simulink model "sampleModel276"  (R2021b)
settings: Solver=VariableStepAuto  StartTime=0.0  StopTime=10.0  RelTol=1e-3
undefined symbols (not defined in the file or in its folder): magnitude
libraries: simulink x8
settings Model: Creator=user  LastModifiedBy=user

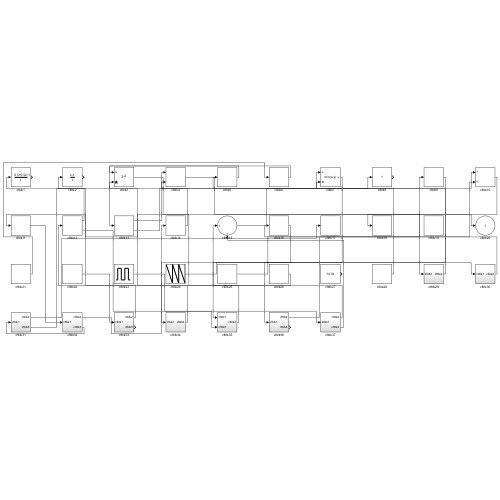
[thumbnail: Simulink's stored preview of the top-level diagram]
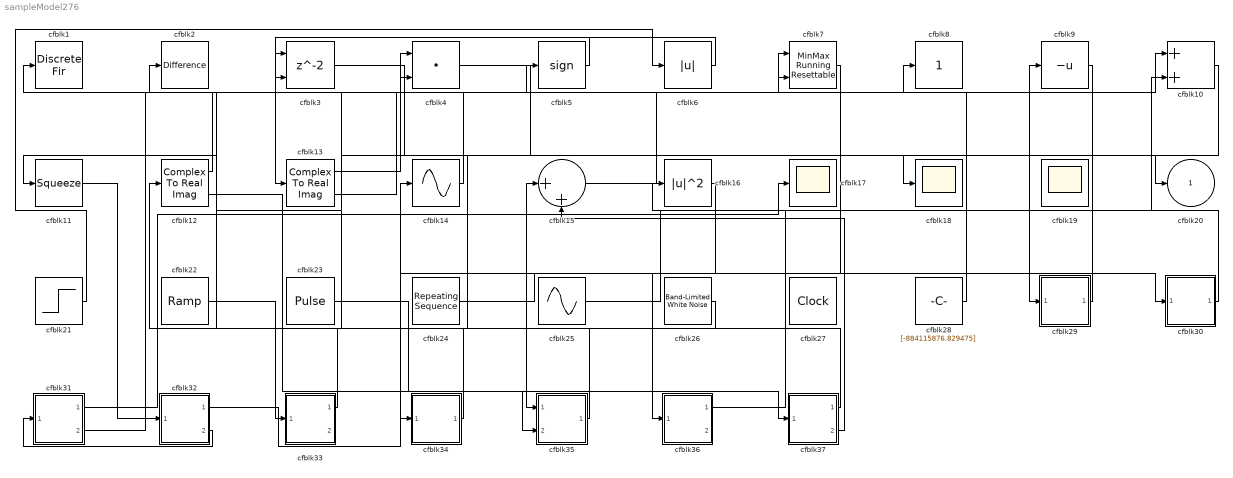
== system sampleModel276 ==
  cfblk1 : DiscreteFir  SampleTime=1
  cfblk10 : Sum
  cfblk11 : Squeeze
  cfblk12 : ComplexToRealImag
  cfblk13 : ComplexToRealImag
  cfblk14 : Sin  TimeSource=Use external signal  SampleTime=0
  cfblk15 : Sum  Inputs=|++
  cfblk16 : Math  Operator=magnitude^2  SaturateOnIntegerOverflow=on
  cfblk17 : Scope
  cfblk18 : Scope
  cfblk19 : Scope
      settings: Floating=on
  cfblk2 : simulink/Discrete/Difference  ICPrevInput=0.0  OutMin=[]  OutMax=[]  OutDataTypeStr=Inherit: Inherit via back propagation  OutDataType=fixdt(1, 16)  OutScaling=2^-10  DoSatur=off
  cfblk21 : Step  Time=[42.000000]  Before=[818983502.483932]  After=[406808043.448474]  SampleTime=0
  cfblk22 : simulink/Sources/Ramp  slope=[-5921.326981]  start=[18.629746]  InitialOutput=[471851.470931]
  cfblk23 : DiscretePulseGenerator  PulseType=Time based  Amplitude=[324430703.930867]  Period=[32077429.850267]  PulseWidth=5  PhaseDelay=[1.000000]
  cfblk24 : simulink/Sources/Repeating Sequence  rep_seq_t=[0 2]  rep_seq_y=[318550818.027670, -776199199.339389]
  cfblk25 : Sin  Amplitude=[-915052577.829016]  Bias=[110707701.179518]  SampleTime=0
  cfblk26 : simulink/Sources/Band-Limited White Noise  Cov=[1529198104.316618]  Ts=0.1  seed=[8998579726.000000]
  cfblk27 : DigitalClock
  cfblk28 : Constant  Value=[-884115876.829475]  SampleTime=1
  cfblk29 : Subsystem
  cfblk3 : Delay  ShowEnablePort=on  SampleTime=1
      settings: InputPortMap=u0,e6
  cfblk30 : Subsystem
  cfblk31 : Subsystem
  cfblk32 : Subsystem
  cfblk33 : Subsystem
  cfblk34 : Subsystem
  cfblk35 : Subsystem
  cfblk36 : Subsystem
  cfblk37 : Subsystem
  cfblk4 : DotProduct  InputSameDT=on  OutDataTypeStr=Inherit: Inherit via internal rule
  cfblk5 : Signum
  cfblk6 : Abs
  cfblk7 : simulink/Math Operations/MinMax Running Resettable  Function=min  vinit=0.0
  cfblk8 : simulink/Math Operations/Slider Gain  gain=1  low=0  high=2
  cfblk9 : UnaryMinus
  cfblk20 : Outport
  wires:
  cfblk4/1 -> cfblk20/1
  cfblk15/1 -> cfblk7/1
  cfblk25/1 -> cfblk9/1
  cfblk5/1 -> cfblk13/1
  cfblk33/1(cfblk2) -> cfblk12/1
  cfblk29/1(cfblk2) -> cfblk7/2
  cfblk32/1(cfblk2) -> cfblk14/1
  cfblk23/1 -> cfblk37/1(cfblk1)
  cfblk26/1 -> cfblk11/1
  cfblk11/1 -> cfblk32/1(cfblk1)
  cfblk12/1 -> cfblk1/1
  cfblk22/1 -> cfblk33/1(cfblk1)
  cfblk32/2(cfblk3) -> cfblk31/1(cfblk1)
  cfblk3/1 -> cfblk29/1(cfblk1)
  cfblk13/1 -> cfblk4/1
  cfblk13/2 -> cfblk10/1
  cfblk37/1(cfblk2) -> cfblk15/1
  cfblk24/1 -> cfblk30/1(cfblk1)
  cfblk21/1 -> cfblk6/1
  cfblk34/1(cfblk2) -> cfblk2/1
  cfblk31/1(cfblk2) -> cfblk17/1
  cfblk16/1 -> cfblk34/1(cfblk1)
  cfblk28/1 -> cfblk5/1
  cfblk14/1 -> cfblk4/2
  cfblk31/2(cfblk4) -> cfblk8/1
  cfblk10/1 -> cfblk18/1
  cfblk30/1(cfblk2) -> cfblk16/1
  cfblk7/1 -> cfblk36/1(cfblk1)
  cfblk9/1 -> cfblk35/1(cfblk1)
  cfblk6/1 -> cfblk3/1
  cfblk12/2 -> cfblk35/2(cfblk5)
  cfblk36/1(cfblk2) -> cfblk10/2
  cfblk37/2(cfblk4) -> cfblk15/2
  cfblk35/1(cfblk2) -> cfblk3/2

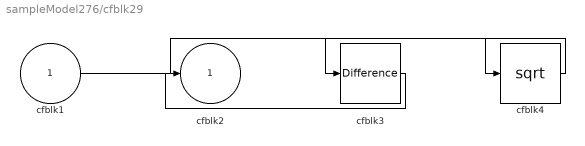
== system sampleModel276/cfblk29 ==
  cfblk1 : Inport
  cfblk3 : simulink/Discrete/Difference  ICPrevInput=0.0  OutMin=[]  OutMax=[]  OutDataTypeStr=Inherit: Inherit via back propagation  OutDataType=fixdt(1, 16)  OutScaling=2^-10  DoSatur=off
  cfblk4 : Sqrt  SaturateOnIntegerOverflow=on
  cfblk2 : Outport
  wires:
  cfblk1/1 -> cfblk4/1
  cfblk3/1 -> cfblk2/1
  cfblk4/1 -> cfblk3/1

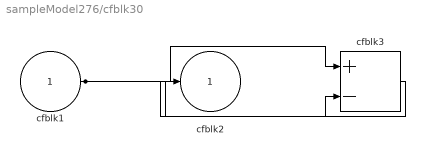
== system sampleModel276/cfblk30 ==
  cfblk1 : Inport
  cfblk3 : Sum  Inputs=+-
  cfblk2 : Outport
  wires:
  cfblk1/1 -> cfblk3/1, cfblk3/2
  cfblk3/1 -> cfblk2/1

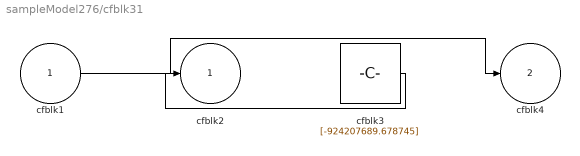
== system sampleModel276/cfblk31 ==
  cfblk1 : Inport
  cfblk3 : Constant  Value=[-924207689.678745]  SampleTime=1
  cfblk2 : Outport
  cfblk4 : Outport  Port=2
  wires:
  cfblk1/1 -> cfblk4/1
  cfblk3/1 -> cfblk2/1

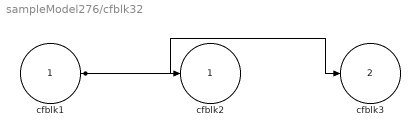
== system sampleModel276/cfblk32 ==
  cfblk1 : Inport
  cfblk2 : Outport
  cfblk3 : Outport  Port=2
  wires:
  cfblk1/1 -> cfblk3/1, cfblk2/1

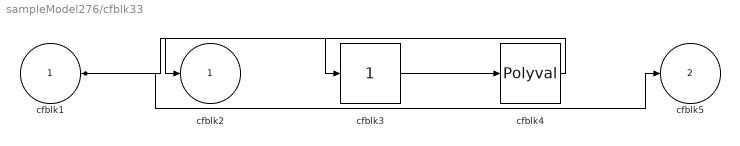
== system sampleModel276/cfblk33 ==
  cfblk1 : Inport
  cfblk3 : simulink/Math Operations/Slider Gain  gain=1  low=0  high=2
  cfblk4 : Polyval  Coefs=[ +2.081618890e-019, -1.441693666e-014, +4.719686976e-010, -8.536869453e-006, +1.621573104e-001, -8.087801117e+001 ]
  cfblk2 : Outport
  cfblk5 : Outport  Port=2
  wires:
  cfblk3/1 -> cfblk4/1
  cfblk4/1 -> cfblk2/1
  cfblk1/1 -> cfblk5/1, cfblk3/1

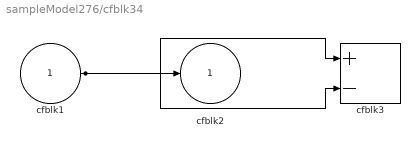
== system sampleModel276/cfblk34 ==
  cfblk1 : Inport
  cfblk3 : Sum  Inputs=+-
  cfblk2 : Outport
  wires:
  cfblk1/1 -> cfblk2/1, cfblk3/1, cfblk3/2

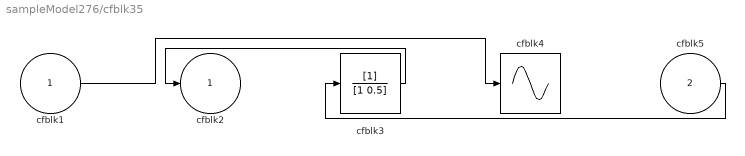
== system sampleModel276/cfblk35 ==
  cfblk1 : Inport
  cfblk5 : Inport  Port=2
  cfblk3 : DiscreteFilter  SampleTime=1
  cfblk4 : Sin  TimeSource=Use external signal  SampleTime=0
  cfblk2 : Outport
  wires:
  cfblk3/1 -> cfblk2/1
  cfblk5/1 -> cfblk3/1
  cfblk1/1 -> cfblk4/1

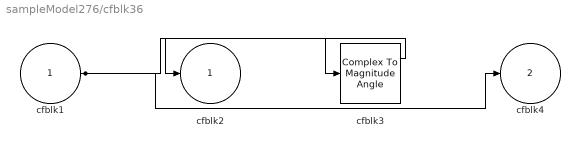
== system sampleModel276/cfblk36 ==
  cfblk1 : Inport
  cfblk3 : ComplexToMagnitudeAngle
  cfblk2 : Outport
  cfblk4 : Outport  Port=2
  wires:
  cfblk3/1 -> cfblk2/1
  cfblk1/1 -> cfblk4/1, cfblk3/1

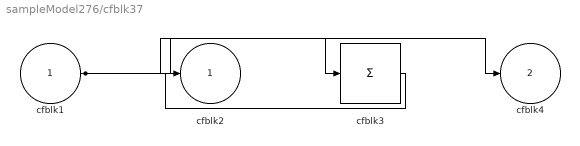
== system sampleModel276/cfblk37 ==
  cfblk1 : Inport
  cfblk3 : Sum  Inputs=+
  cfblk2 : Outport
  cfblk4 : Outport  Port=2
  wires:
  cfblk1/1 -> cfblk4/1, cfblk3/1
  cfblk3/1 -> cfblk2/1
